simulink model "getDataSim"  (R2013a)
settings: Solver=ode45  StartTime=0.0  StopTime=t  RelTol=1e-3
values from neighbouring files (symbols this model uses):
  sampleTimeCam = 0.0161    [runMySystem.m]
undefined symbols (not defined in the file or in its folder): sampleTime
libraries: aerolibutil x1
settings Model: Creator=User  LastModifiedBy=User

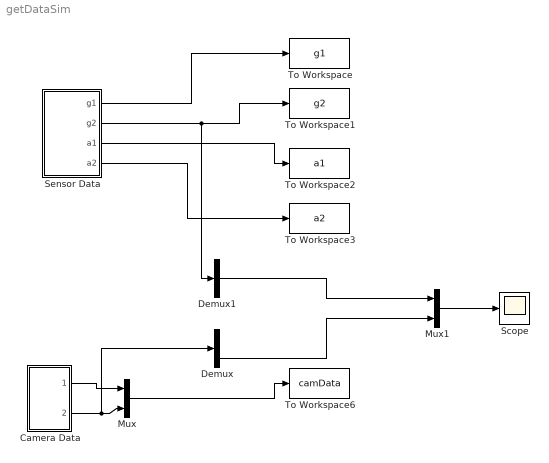
== system getDataSim ==
  Camera Data : Subsystem
  Demux : Demux  Outputs=3
  Demux1 : Demux  Outputs=3
  Mux : Mux  Inputs=2
  Mux1 : Mux  Inputs=2
  Scope : Scope
      settings: SaveName=ScopeData6
  Sensor Data : Subsystem
  To Workspace : ToWorkspace  VariableName=g1  SampleTime=sampleTime  SaveFormat=Structure With Time
  To Workspace1 : ToWorkspace  VariableName=g2  SampleTime=sampleTime  SaveFormat=Structure With Time
  To Workspace2 : ToWorkspace  VariableName=a1  SampleTime=sampleTime  SaveFormat=Structure With Time
  To Workspace3 : ToWorkspace  VariableName=a2  SampleTime=sampleTime  SaveFormat=Structure With Time
  To Workspace6 : ToWorkspace  VariableName=camData  SampleTime=sampleTime  SaveFormat=Structure With Time
  wires:
  Sensor Data/1("g1 ") -> To Workspace/1
  Sensor Data/2("g2 ") -> Demux1/1, To Workspace1/1
  Sensor Data/3(a1) -> To Workspace2/1
  Sensor Data/4(a2) -> To Workspace3/1
  Mux/1 -> To Workspace6/1
  Camera Data/1(camS1) -> Mux/1
  Camera Data/2(camS2) -> Demux/1, Mux/2
  Demux1/2 -> Mux1/1
  Demux/3 -> Mux1/2
  Mux1/1 -> Scope/1

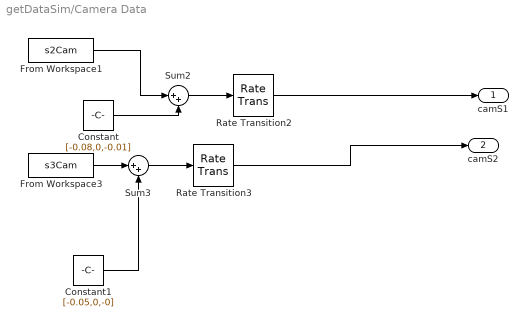
== system getDataSim/Camera Data ==
  Constant : Constant  Value=[-0.08,0,-0.01]
  Constant1 : Constant  Value=[-0.05,0,-0]
  From Workspace1 : FromWorkspace  VariableName=s2Cam  SampleTime=sampleTimeCam
  From Workspace3 : FromWorkspace  VariableName=s3Cam  SampleTime=sampleTimeCam
  Rate Transition2 : RateTransition  Deterministic=off
  Rate Transition3 : RateTransition  Deterministic=off
  Sum2 : Sum  Inputs=|++
  Sum3 : Sum  Inputs=|++
  camS1 : Outport
  camS2 : Outport  Port=2
  wires:
  Sum3/1 -> Rate Transition3/1
  From Workspace1/1 -> Sum2/1
  Constant/1 -> Sum2/2
  Rate Transition2/1 -> camS1/1
  Constant1/1 -> Sum3/2
  Sum2/1 -> Rate Transition2/1
  From Workspace3/1 -> Sum3/1
  Rate Transition3/1 -> camS2/1

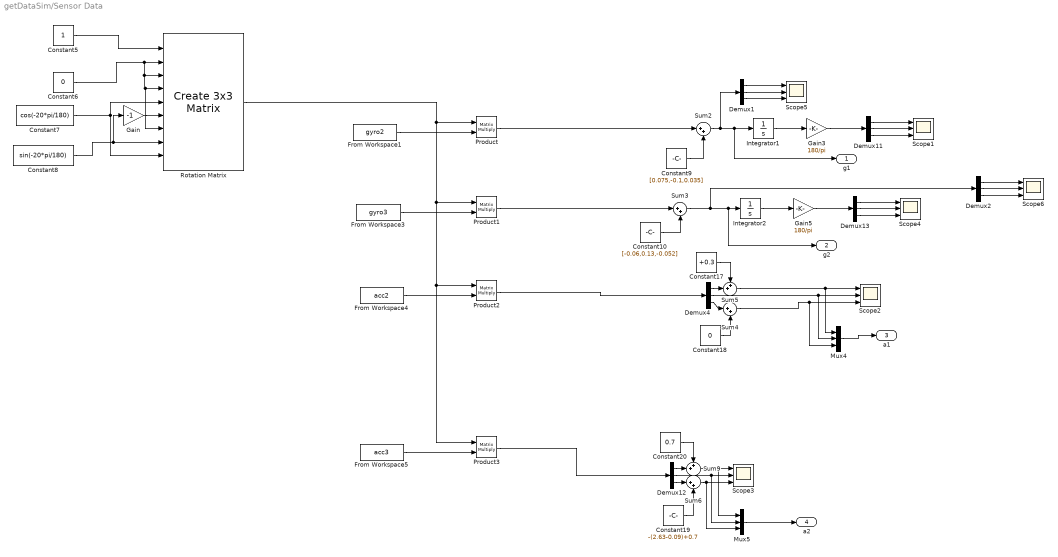
== system getDataSim/Sensor Data ==
  Constant10 : Constant  Value=[-0.06,0.13,-0.052]
  Constant17 : Constant  Value=+0.3
  Constant18 : Constant  Value=0
  Constant19 : Constant  Value=-(2.63-0.09)+0.7
  Constant20 : Constant  Value=0.7
  Constant5 : Constant
  Constant6 : Constant  Value=0
  Constant7 : Constant  Value=cos(-20*pi/180)
  Constant8 : Constant  Value=sin(-20*pi/180)
  Constant9 : Constant  Value=[0.075,-0.1,0.035]
  Demux{1..2,4,11..13} (6 alike) : Demux  Outputs=3
  From Workspace1 : FromWorkspace  VariableName=gyro2  SampleTime=sampleTime
  From Workspace3 : FromWorkspace  VariableName=gyro3  SampleTime=sampleTime
  From Workspace4 : FromWorkspace  VariableName=acc2  SampleTime=sampleTime
  From Workspace5 : FromWorkspace  VariableName=acc3  SampleTime=sampleTime
  Gain : Gain  Gain=-1
  Gain3 : Gain  Gain=180/pi
  Gain5 : Gain  Gain=180/pi
  Integrator1 : Integrator
  Integrator2 : Integrator
  Mux4 : Mux  Inputs=3
  Mux5 : Mux  Inputs=3
  Product{,1..3} (4 alike) : Product  Multiplication=Matrix(*)
  Rotation Matrix : aerolibutil/Create 3x3 Matrix
  Scope{1..6} (6 alike) : Scope  NumInputPorts=3
      Scope1 settings: TimeRange=6  YMin=-35~-35~-35  YMax=0~5~5
      Scope2 settings: YMin=-5~-5~-5  YMax=5~5~5
      Scope3 settings: YMin=-5~-5~-5  YMax=5~5~5  SaveName=ScopeData2
      Scope4 settings: YMin=-5~-5~-5  YMax=5~5~5  SaveName=ScopeData3
      Scope5 settings: TimeRange=6  YMin=-35~-35~-35  YMax=0~5~5  SaveName=ScopeData4
      Scope6 settings: TimeRange=6  YMin=-35~-35~-35  YMax=0~5~5  SaveName=ScopeData5
  Sum{2..4,6} (4 alike) : Sum  Inputs=|++
  Sum5 : Sum  Inputs=++|
  Sum9 : Sum  Inputs=++|
  "g1 " : Outport
  "g2 " : Outport  Port=2
  a1 : Outport  Port=3
  a2 : Outport  Port=4
  wires:
  Constant5/1 -> Rotation Matrix/1
  Constant6/1 -> Rotation Matrix/7, Rotation Matrix/4, Rotation Matrix/3, Rotation Matrix/2
  Constant7/1 -> Rotation Matrix/5, Rotation Matrix/9
  Constant8/1 -> Gain/1, Rotation Matrix/8
  Gain/1 -> Rotation Matrix/6
  From Workspace1/1 -> Product/2
  From Workspace3/1 -> Product1/2
  From Workspace4/1 -> Product2/2
  From Workspace5/1 -> Product3/2
  Rotation Matrix/1 -> Product3/1, Product2/1, Product1/1, Product/1
  Integrator1/1 -> Gain3/1
  Demux11/1 -> Scope1/1
  Demux11/2 -> Scope1/2
  Demux11/3 -> Scope1/3
  Gain3/1 -> Demux11/1
  Constant9/1 -> Sum2/2
  Demux13/1 -> Scope4/1
  Demux13/2 -> Scope4/2
  Demux13/3 -> Scope4/3
  Integrator2/1 -> Gain5/1
  Gain5/1 -> Demux13/1
  Product1/1 -> Sum3/1
  Constant10/1 -> Sum3/2
  Product2/1 -> Demux4/1
  Sum5/1 -> Mux4/1, Scope2/1
  Demux4/2 -> Mux4/2, Scope2/2
  Sum4/1 -> Mux4/3, Scope2/3
  Demux4/3 -> Sum4/1
  Constant18/1 -> Sum4/2
  Demux4/1 -> Sum5/2
  Constant17/1 -> Sum5/1
  Mux4/1 -> a1/1
  Product3/1 -> Demux12/1
  Sum9/1 -> Mux5/1, Scope3/1
  Demux12/2 -> Mux5/2, Scope3/2
  Sum6/1 -> Mux5/3, Scope3/3
  Demux12/3 -> Sum6/1
  Constant19/1 -> Sum6/2
  Demux12/1 -> Sum9/2
  Constant20/1 -> Sum9/1
  Mux5/1 -> a2/1
  Demux1/1 -> Scope5/1
  Demux1/2 -> Scope5/2
  Demux1/3 -> Scope5/3
  Sum2/1 -> Demux1/1, "g1 "/1, Integrator1/1
  Product/1 -> Sum2/1
  Demux2/1 -> Scope6/1
  Demux2/2 -> Scope6/2
  Demux2/3 -> Scope6/3
  Sum3/1 -> Demux2/1, "g2 "/1, Integrator2/1
